simulink model "BlueROVHeavy_FeedbackLinearizationControl"  (R2024b)
settings: Solver=ode45  StartTime=0.0  StopTime=T  MaxStep=0.01  RelTol=1e-3
InitFcn:
  | run BlueRovHeavy_init.m;
StopFcn:
  | run BlueRovHeavy_plotting.m;
values from neighbouring files (symbols this model uses):
  BLUEROV_DATA = struct()    [BlueRovHeavy_data.m]
  Kf_D = 43    [BlueRovHeavy_init.m]
  Kf_P = 78    [BlueRovHeavy_init.m]
libraries: robotcorelib x1
settings Model: Creator=salva  LastModifiedBy=salva

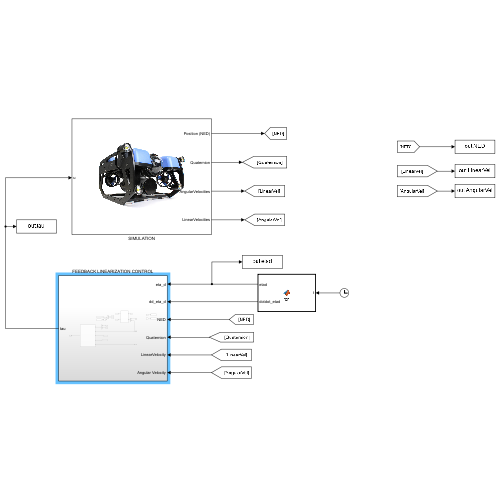
[thumbnail: Simulink's stored preview of the top-level diagram]
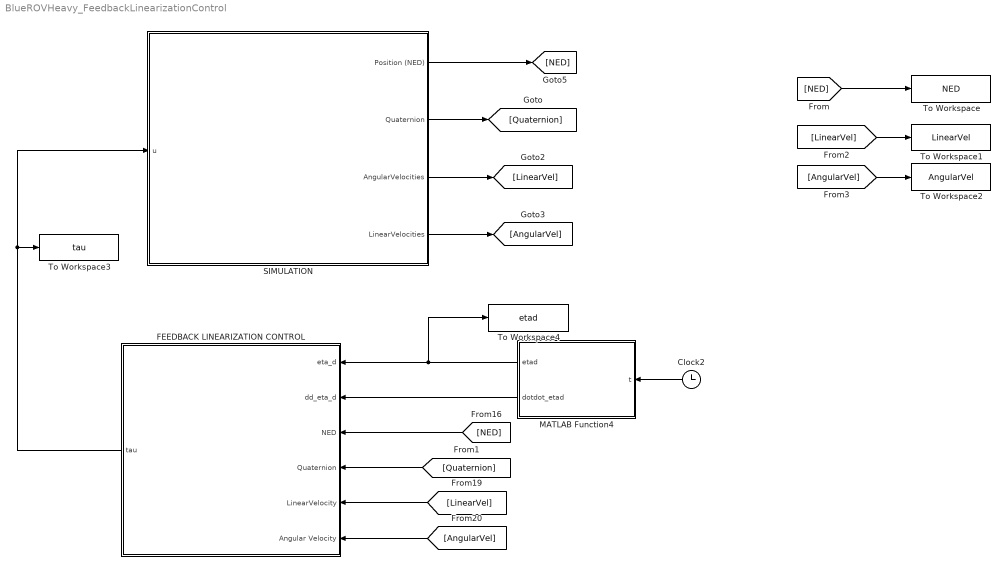
== system BlueROVHeavy_FeedbackLinearizationControl ==
  Clock2 : Clock
  FEEDBACK LINEARIZATION CONTROL : Subsystem
  MATLAB Function4 : MATLAB Function  TreatAsAtomicUnit=on
  SIMULATION : Subsystem
      mask Display: image('BlueROVpic.jpg', [0,0,0,0,90,90]);
  To Workspace : ToWorkspace  VariableName=NED  SaveFormat=Timeseries  SampleTime=-1
  To Workspace1 : ToWorkspace  VariableName=LinearVel  SaveFormat=Timeseries  SampleTime=-1
  To Workspace2 : ToWorkspace  VariableName=AngularVel  SaveFormat=Timeseries  SampleTime=-1
  To Workspace3 : ToWorkspace  VariableName=tau  SaveFormat=Timeseries  SampleTime=-1
  To Workspace4 : ToWorkspace  VariableName=etad  SaveFormat=Timeseries  SampleTime=-1
  wires:
  SIMULATION/1(Position (NED)) -> [NED]
  SIMULATION/2(Quaternion) -> [Quaternion]
  SIMULATION/3(AngularVelocities) -> [LinearVel]
  SIMULATION/4(LinearVelocities) -> [AngularVel]
  Clock2/1 -> MATLAB Function4/1(t)
  [LinearVel] -> FEEDBACK LINEARIZATION CONTROL/5(LinearVelocity)
  [AngularVel] -> FEEDBACK LINEARIZATION CONTROL/6(Angular Velocity)
  [Quaternion] -> FEEDBACK LINEARIZATION CONTROL/4(Quaternion)
  FEEDBACK LINEARIZATION CONTROL/1(tau) -> SIMULATION/1(u), To Workspace3/1
  MATLAB Function4/1(etad) -> To Workspace4/1, FEEDBACK LINEARIZATION CONTROL/1(eta_d)
  [NED] -> FEEDBACK LINEARIZATION CONTROL/3(NED)
  MATLAB Function4/2(dotdot_etad) -> FEEDBACK LINEARIZATION CONTROL/2(dd_eta_d)
  [NED] -> To Workspace/1
  [LinearVel] -> To Workspace1/1
  [AngularVel] -> To Workspace2/1

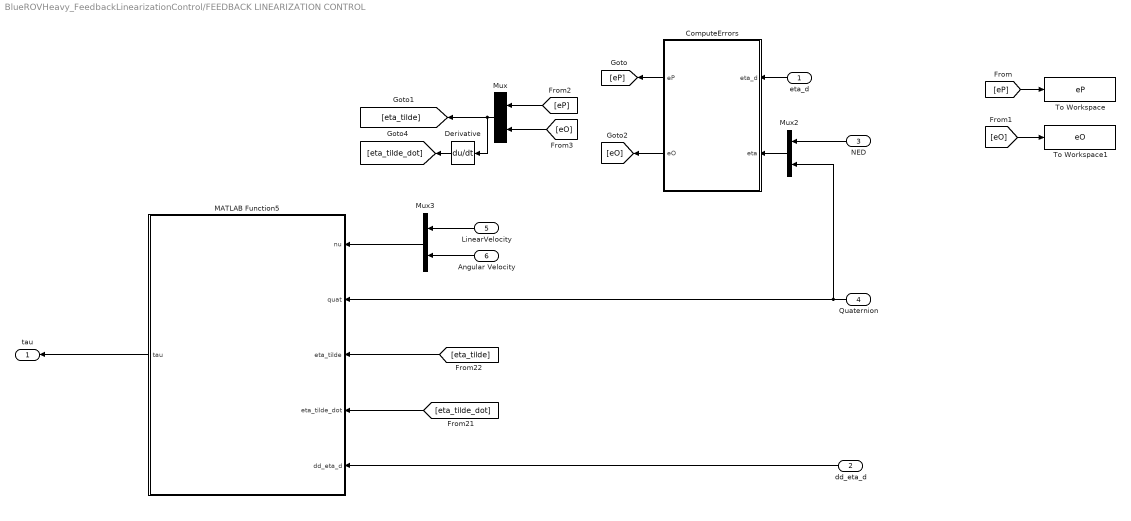
== system BlueROVHeavy_FeedbackLinearizationControl/FEEDBACK LINEARIZATION CONTROL ==
  eta_d : Inport
  dd_eta_d : Inport  Port=2
  NED : Inport  Port=3
  Quaternion : Inport  Port=4
  LinearVelocity : Inport  Port=5
  Angular Velocity : Inport  Port=6
  ComputeErrors : MATLAB Function  TreatAsAtomicUnit=on
  Derivative : Derivative
  MATLAB Function5 : MATLAB Function  TreatAsAtomicUnit=on
  Mux : Mux  Inputs=2
  Mux2 : Mux  Inputs=2
  Mux3 : Mux  Inputs=2
  To Workspace : ToWorkspace  VariableName=eP  SaveFormat=Timeseries  SampleTime=-1
  To Workspace1 : ToWorkspace  VariableName=eO  SaveFormat=Timeseries  SampleTime=-1
  tau : Outport
  wires:
  [eta_tilde_dot] -> MATLAB Function5/4(eta_tilde_dot)
  Mux2/1 -> ComputeErrors/2(eta)
  [eta_tilde] -> MATLAB Function5/3(eta_tilde)
  Mux3/1 -> MATLAB Function5/1(nu)
  LinearVelocity/1 -> Mux3/1
  Angular Velocity/1 -> Mux3/2
  MATLAB Function5/1(tau) -> tau/1
  NED/1 -> Mux2/1
  dd_eta_d/1 -> MATLAB Function5/5(dd_eta_d)
  eta_d/1 -> ComputeErrors/1(eta_d)
  Quaternion/1 -> MATLAB Function5/2(quat), Mux2/2
  Derivative/1 -> [eta_tilde_dot]
  Mux/1 -> [eta_tilde], Derivative/1
  ComputeErrors/1(eP) -> [eP]
  ComputeErrors/2(eO) -> [eO]
  [eP] -> To Workspace/1
  [eP] -> Mux/1
  [eO] -> Mux/2
  [eO] -> To Workspace1/1

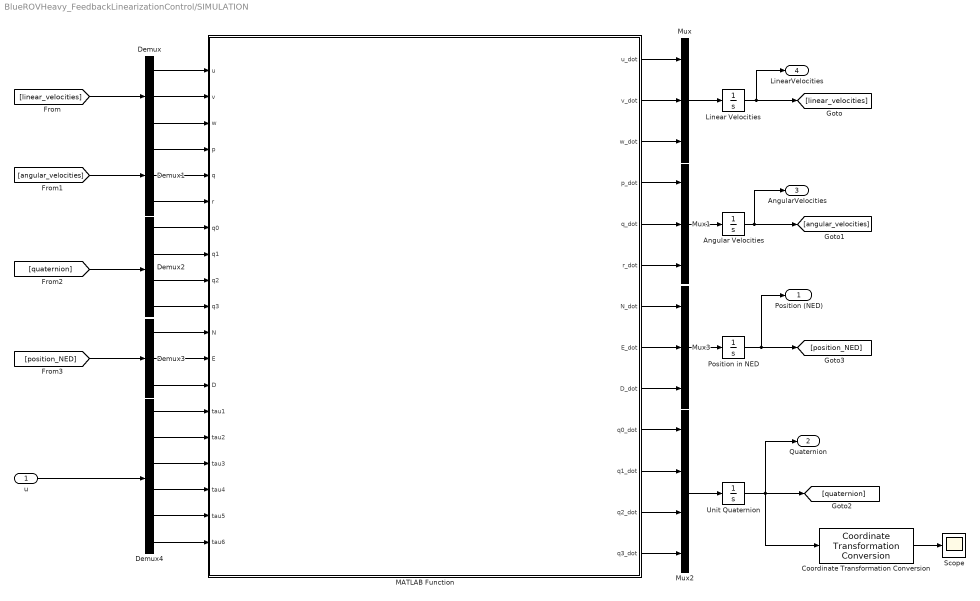
== system BlueROVHeavy_FeedbackLinearizationControl/SIMULATION ==
  u : Inport
  Angular Velocities : Integrator  InitialCondition=[0;0;0]  UpperSaturationLimit=50  LowerSaturationLimit=-50
  Coordinate Transformation Conversion : robotcorelib/Coordinate Transformation Conversion  InputRepresentation=Quaternion  InputEulerSequence=ZYX  ShowTrVecInputPort=on  OutputRepresentation=Euler Angles  OutputEulerSequence=XYZ  ShowTrVecOutputPort=on  SimulateUsing=Interpreted execution
  Demux : Demux  Outputs=3
  Demux1 : Demux  Outputs=3
  Demux2 : Demux
  Demux3 : Demux  Outputs=3
  Demux4 : Demux  Outputs=6
  Linear Velocities : Integrator  InitialCondition=[0.1;0;0]
  MATLAB Function : MATLAB Function  TreatAsAtomicUnit=on
  Mux : Mux  Inputs=3
  Mux1 : Mux  Inputs=3
  Mux2 : Mux
  Mux3 : Mux  Inputs=3
  Position in NED : Integrator  InitialCondition=[3.5;0;9.5]
  Scope : Scope
  Unit Quaternion : Integrator  InitialCondition=[1,0,0,0]
  Position (NED) : Outport
  Quaternion : Outport  Port=2
  AngularVelocities : Outport  Port=3
  LinearVelocities : Outport  Port=4
  wires:
  Demux/3 -> MATLAB Function/3(w)
  MATLAB Function/5(q_dot) -> Mux1/2
  Demux1/1 -> MATLAB Function/4(p)
  MATLAB Function/6(r_dot) -> Mux1/3
  Demux3/2 -> MATLAB Function/12(E)
  MATLAB Function/7(N_dot) -> Mux3/1
  Mux1/1 -> Angular Velocities/1
  Demux2/2 -> MATLAB Function/8(q1)
  MATLAB Function/2(v_dot) -> Mux/2
  Demux4/1 -> MATLAB Function/14(tau1)
  Demux3/3 -> MATLAB Function/13(D)
  Mux2/1 -> Unit Quaternion/1
  Demux4/4 -> MATLAB Function/17(tau4)
  Demux4/5 -> MATLAB Function/18(tau5)
  MATLAB Function/1(u_dot) -> Mux/1
  MATLAB Function/11(q1_dot) -> Mux2/2
  MATLAB Function/3(w_dot) -> Mux/3
  MATLAB Function/12(q2_dot) -> Mux2/3
  Demux3/1 -> MATLAB Function/11(N)
  MATLAB Function/4(p_dot) -> Mux1/1
  MATLAB Function/9(D_dot) -> Mux3/3
  [linear_velocities] -> Demux/1
  Demux4/3 -> MATLAB Function/16(tau3)
  u/1 -> Demux4/1
  Demux1/2 -> MATLAB Function/5(q)
  Mux/1 -> Linear Velocities/1
  Demux2/3 -> MATLAB Function/9(q2)
  [quaternion] -> Demux2/1
  Demux/1 -> MATLAB Function/1(u)
  Demux4/2 -> MATLAB Function/15(tau2)
  MATLAB Function/13(q3_dot) -> Mux2/4
  Demux2/4 -> MATLAB Function/10(q3)
  Mux3/1 -> Position in NED/1
  Demux2/1 -> MATLAB Function/7(q0)
  Unit Quaternion/1 -> Coordinate Transformation Conversion/1, Quaternion/1, [quaternion]
  Demux4/6 -> MATLAB Function/19(tau6)
  Position in NED/1 -> Position (NED)/1, [position_NED]
  Demux1/3 -> MATLAB Function/6(r)
  MATLAB Function/10(q0_dot) -> Mux2/1
  Angular Velocities/1 -> [angular_velocities], AngularVelocities/1
  [angular_velocities] -> Demux1/1
  Linear Velocities/1 -> [linear_velocities], LinearVelocities/1
  Demux/2 -> MATLAB Function/2(v)
  [position_NED] -> Demux3/1
  Coordinate Transformation Conversion/1 -> Scope/1
  MATLAB Function/8(E_dot) -> Mux3/2

== matlab function BlueROVHeavy_FeedbackLinearizationControl/FEEDBACK LINEARIZATION CONTROL/MATLAB Function5 ==
  data: nu input; tau output; quat input; eta_tilde input; eta_tilde_dot input; dd_eta_d input; BLUEROV_DATA parameter; Kf_D parameter; Kf_P parameter
function tau = fcn(nu,quat,eta_tilde,eta_tilde_dot,dd_eta_d, BLUEROV_DATA, Kf_D, Kf_P)

    u=nu(1);
    v=nu(2);
    w=nu(3);
    p=nu(4);
    q=nu(5);
    r=nu(6);
    q0=quat(1);
    q1=quat(2);
    q2=quat(3);
    q3=quat(4);




    % dq0=dotquat(1);
    % dq1=dotquat(2);
    % dq2=dotquat(3);
    % dq3=dotquat(4);
    Omega = 0.5 * [
     0   -p   -q  -r;
     p    0    r  -q;
     q  -r    0   p;
     r    q  -p   0
    ];

    dq= Omega*quat;
    dq0=dq(1);
    dq1=dq(2);
    dq2=dq(3);
    dq3=dq(4);





    e1 = BLUEROV_DATA.e1;                    %Body frame unit vector along x
    e2 = BLUEROV_DATA.e2;                    %Body frame unit vector along y
    e3 = BLUEROV_DATA.e3;                    %Body frame unit vector along z
    
    I3 = BLUEROV_DATA.I3;                      %Identity matrix (3x3)
    
    
    m_t = BLUEROV_DATA.m_t;                      %BlueROV mass [Kg]
    W = BLUEROV_DATA.W;                       %Weight [N]
    B = BLUEROV_DATA.B;                       %Boyancy [N]
    r_cb = BLUEROV_DATA.r_cb;                 %Center of boyancy wrt. center of origin [m]
    r_cg = BLUEROV_DATA.r_cg;                %Center of gravity wrt. center of origin [m]
    
    I = BLUEROV_DATA.I;                     %Dyadyic inertia
    SCG =BLUEROV_DATA.SCG;
    
    
    %% Added mass (hydrodynamic derivatives)
    
    X_udot = BLUEROV_DATA.X_udot;   % [kg] 
    Y_vdot = BLUEROV_DATA.Y_vdot;  % [kg]
    Z_wdot = BLUEROV_DATA.Z_wdot; % [kg]
    K_pdot = BLUEROV_DATA.K_pdot;  % [kg m^2/rad]
    M_qdot = BLUEROV_DATA.M_qdot;  % [kg m^2/rad]
    N_rdot = BLUEROV_DATA.N_rdot;  % [kg m^2/rad]
    
    %% Hydrodynamic linear and quadratic damping coefficients
    
    Xu = BLUEROV_DATA.Xu;      % [Ns/m]
    Yv = BLUEROV_DATA.Yv;      % [Ns/m]
    Zw = BLUEROV_DATA.Zw;      % [Ns/m]
    Kp = BLUEROV_DATA.Kp;      % [Ns/rad]
    Mq = BLUEROV_DATA.Mq;      % [Ns/rad]
    Nr = BLUEROV_DATA.Nr;      % [Ns/rad]
    
    Xuu = BLUEROV_DATA.Xuu;    % [Ns^2/m^2]
    Yvv = BLUEROV_DATA.Yvv;    % [Ns^2/m^2]
    Zww = BLUEROV_DATA.Zww;    % [Ns^2/m^2]
    Kpp = BLUEROV_DATA.Kpp;     % [Ns^2/rad^2]
    Mqq = BLUEROV_DATA.Mqq;     % [Ns^2/rad^2]
    Nrr = BLUEROV_DATA.Nrr;     % [Ns^2/rad^2]
        
    %% Kinematics
    
    Rq=[1-2*(q2^2+q3^2) 2*(q1*q2-q3*q0) 2*(q1*q3+q2*q0);
        2*(q1*q2+q3*q0) 1-2*(q1^2+q3^2) 2*(q2*q3-q1*q0);
        2*(q1*q3-q2*q0) 2*(q2*q3+q1*q0) 1-2*(q1^2+q2^2)];
    Tq=0.5*[-q1,-q2,-q3;
        q0,-q3,q2;
        q3,q0,-q1;
        -q2,q1,q0];

    J_qeta=[Rq,zeros(3,3);zeros(4,3),Tq];


 
    %% Computing Hydrodynamic Damping Matrix D(v)
    epsilon=1e-4;

    D = diag([Xu + Xuu*sqrt(u^2 + epsilon), ...
          Yv + Yvv*sqrt(v^2 + epsilon), ...
          Zw + Zww*sqrt(w^2 + epsilon), ...
          Kp + Kpp*sqrt(p^2 + epsilon), ...
          Mq + Mqq*sqrt(q^2 + epsilon), ...
          Nr + Nrr*sqrt(r^2 + epsilon)]);


    %% Computing Restoring Forces
    
    g_eta = [(-W+B)*(2*q1*q3-2*q2*q0);
            -(W-B)*(2*q2*q3-2*q1*q0);
            (W-B)*(2*q1^2+2*q2^2-1);
            r_cg(3)*W*(2*q2*q3+2*q1*q0);
            r_cg(3)*W*(2*q1*q3-2*q2*q0);
            0];
    
   
    %% Computing Coriolis and Centrifugal Matrix C(v)
     IO = I*[p q r]'; 
     
     S_IO = [0 -IO(3) IO(2);
             IO(3) 0 -IO(1);
            -IO(2) IO(1) 0]; 
             
    S_omega = [0 -r q;
              r 0 -p;
              -q p 0];         
             
       
    C_rb = [m_t*S_omega -m_t*S_omega*SCG;
            m_t*SCG*S_omega -S_IO];
        
    
    C_A = [0 0 0 0 -Z_wdot*w Y_vdot*v;
           0 0 0 -Z_wdot*w 0 -X_udot*u;
           0 0 0 -Y_vdot*v X_udot*u 0;
           0 -Z_wdot*w Y_vdot*v 0 -N_rdot*r M_qdot*q;
           Z_wdot*w 0 -X_udot*u N_rdot*r 0 -K_pdot*p;
           -Y_vdot*v X_udot*u 0 -M_qdot*q K_pdot*p 0];

    Cv=C_rb+C_A;

    %% Total Inertia
    M=BLUEROV_DATA.M;
    

    pinvJ_qeta=pinv(J_qeta); % Moonre_Penrose Inverse of the jacobian (since we are using quaternions)
    
    Jdot=compute_Jdot(q0,q1,q2,q3,dq0,dq1,dq2,dq3);%Jacobian derivative

    n=(Cv+D)*[u v w p q r]'+g_eta;

    lambda_n=dd_eta_d+Kf_D*eta_tilde_dot+Kf_P*eta_tilde;
    lambda_b=pinvJ_qeta*(lambda_n-Jdot*nu);

    tau=n+M*lambda_b;

== matlab function BlueROVHeavy_FeedbackLinearizationControl/SIMULATION/MATLAB Function ==
  data: u input; u_dot output; v input; w input; p input; q input; r input; q0 input; q1 input; q2 input; q3 input; N input; E input; D input; tau1 input; tau2 input; tau3 input; tau4 input; tau5 input; tau6 input; v_dot output; w_dot output; p_dot output; q_dot output; r_dot output; N_dot output; E_dot output; D_dot output; q0_dot output; q1_dot output; q2_dot output; q3_dot output; BLUEROV_DATA parameter

function [u_dot, v_dot, w_dot, p_dot, q_dot, r_dot,N_dot,E_dot,D_dot, q0_dot,q1_dot,q2_dot,q3_dot] =  ...
    BlueROV(u, v, w, p, q, r, q0,q1,q2,q3, N, E, D, tau1,tau2,tau3,tau4,tau5,tau6, BLUEROV_DATA)
    
    e1 = BLUEROV_DATA.e1;                    %Body frame unit vector along x
    e2 = BLUEROV_DATA.e2;                    %Body frame unit vector along y
    e3 = BLUEROV_DATA.e3;                    %Body frame unit vector along z
    
    I3 = BLUEROV_DATA.I3;                      %Identity matrix (3x3)
    
    
    m_t = BLUEROV_DATA.m_t;                      %BlueROV mass [Kg]
    W = BLUEROV_DATA.W;                       %Weight [N]
    B = BLUEROV_DATA.B;                       %Boyancy [N]
    r_cb = BLUEROV_DATA.r_cb;                 %Center of boyancy wrt. center of origin [m]
    r_cg = BLUEROV_DATA.r_cg;                %Center of gravity wrt. center of origin [m]
    
    I = BLUEROV_DATA.I;                     %Dyadyic inertia
    SCG =BLUEROV_DATA.SCG;
    
    
    %% Added mass (hydrodynamic derivatives)
    
    X_udot = BLUEROV_DATA.X_udot;   % [kg] 
    Y_vdot = BLUEROV_DATA.Y_vdot;  % [kg]
    Z_wdot = BLUEROV_DATA.Z_wdot; % [kg]
    K_pdot = BLUEROV_DATA.K_pdot;  % [kg m^2/rad]
    M_qdot = BLUEROV_DATA.M_qdot;  % [kg m^2/rad]
    N_rdot = BLUEROV_DATA.N_rdot;  % [kg m^2/rad]
    
    %% Hydrodynamic linear and quadratic damping coefficients
    
    Xu = BLUEROV_DATA.Xu;      % [Ns/m]
    Yv = BLUEROV_DATA.Yv;      % [Ns/m]
    Zw = BLUEROV_DATA.Zw;      % [Ns/m]
    Kp = BLUEROV_DATA.Kp;      % [Ns/rad]
    Mq = BLUEROV_DATA.Mq;      % [Ns/rad]
    Nr = BLUEROV_DATA.Nr;      % [Ns/rad]
    
    Xuu = BLUEROV_DATA.Xuu;    % [Ns^2/m^2]
    Yvv = BLUEROV_DATA.Yvv;    % [Ns^2/m^2]
    Zww = BLUEROV_DATA.Zww;    % [Ns^2/m^2]
    Kpp = BLUEROV_DATA.Kpp;     % [Ns^2/rad^2]
    Mqq = BLUEROV_DATA.Mqq;     % [Ns^2/rad^2]
    Nrr = BLUEROV_DATA.Nrr;     % [Ns^2/rad^2]
    
    
    
    %% Kinematics
    
    Rq=[1-2*(q2^2+q3^2) 2*(q1*q2-q3*q0) 2*(q1*q3+q2*q0);
        2*(q1*q2+q3*q0) 1-2*(q1^2+q3^2) 2*(q2*q3-q1*q0);
        2*(q1*q3-q2*q0) 2*(q2*q3+q1*q0) 1-2*(q1^2+q2^2)];
    Tq=0.5*[-q1,-q2,-q3;
        q0,-q3,q2;
        q3,q0,-q1;
        -q2,q1,q0];

    J_qeta=[Rq,zeros(3,3);zeros(4,3),Tq];
 
    %% Computing Hydrodynamic Damping Matrix D(v)
    epsilon=1e-4;

    D = diag([Xu + Xuu*sqrt(u^2 + epsilon), ...
          Yv + Yvv*sqrt(v^2 + epsilon), ...
          Zw + Zww*sqrt(w^2 + epsilon), ...
          Kp + Kpp*sqrt(p^2 + epsilon), ...
          Mq + Mqq*sqrt(q^2 + epsilon), ...
          Nr + Nrr*sqrt(r^2 + epsilon)]);


    %% Computing Restoring Forces
    
    g_eta = [(-W+B)*(2*q1*q3-2*q2*q0);
            -(W-B)*(2*q2*q3-2*q1*q0);
            (W-B)*(2*q1^2+2*q2^2-1);
            r_cg(3)*W*(2*q2*q3+2*q1*q0);
            r_cg(3)*W*(2*q1*q3-2*q2*q0);
            0];
    
   
    %% Computing Coriolis and Centrifugal Matrix C(v)
     IO = I*[p q r]'; 
     
     S_IO = [0 -IO(3) IO(2);
             IO(3) 0 -IO(1);
            -IO(2) IO(1) 0]; 
             
    S_omega = [0 -r q;
              r 0 -p;
              -q p 0];         
             
       
    C_rb = [m_t*S_omega -m_t*S_omega*SCG;
            m_t*SCG*S_omega -S_IO];
        
    
    C_A = [0 0 0 0 -Z_wdot*w Y_vdot*v;
           0 0 0 -Z_wdot*w 0 -X_udot*u;
           0 0 0 -Y_vdot*v X_udot*u 0;
           0 -Z_wdot*w Y_vdot*v 0 -N_rdot*r M_qdot*q;
           Z_wdot*w 0 -X_udot*u N_rdot*r 0 -K_pdot*p;
           -Y_vdot*v X_udot*u 0 -M_qdot*q K_pdot*p 0];
        
    %% Generalized forces and moments
    tau_c = [tau1 tau2 tau3 tau4 tau5 tau6]';

    %% Total Inertia Matric
    M=BLUEROV_DATA.M;


    %% 6DOF Dynamics and Kinematics
    
    nu_dot=zeros(6,1);
    nu_dot = M\(tau_c-(D+C_rb+C_A)*[u v w p q r]' -g_eta); %6DOF dynamics

    etadot=zeros(7,1); 
    etadot=J_qeta*[u v w p q r]'; %Kinematics
    
    u_dot = nu_dot(1); %Surge velcoity
    v_dot = nu_dot(2); %Sway Velcoity
    w_dot = nu_dot(3); %Heave velocity
    p_dot = nu_dot(4); %Angular velocity around phi
    q_dot = nu_dot(5);  %Angular velcoity around theta
    r_dot = nu_dot(6); %Angular velcoity around psi
  
   
    
    N_dot=etadot(1); % N position
    E_dot=etadot(2); % E position
    D_dot=etadot(3); % D position
    q0_dot=etadot(4); % Quaternion
    q1_dot=etadot(5);
    q2_dot=etadot(6);
    q3_dot=etadot(7);

== matlab function BlueROVHeavy_FeedbackLinearizationControl/FEEDBACK LINEARIZATION CONTROL/ComputeErrors ==
  data: eP output; eta_d input; eO output; eta input
function [eP,eO] = fcn(eta_d,eta)

Qd=eta_d(4:7);
Qe=eta(4:7);

Sd=[0 -Qd(4) Qd(3);
    Qd(4) 0 -Qd(2);
    -Qd(3) Qd(2) 0];

eO=[Qd(1)*Qe(1)+Qd(2:4)'*Qe(2:4);Qe(1)*Qd(2:4)-Qd(1)*Qe(2:4)-Sd*Qe(2:4)];

eP=eta_d(1:3)-eta(1:3);

== matlab function BlueROVHeavy_FeedbackLinearizationControl/MATLAB Function4 ==
  data: t input; etad output; dotdot_etad output
function [etad,dotdot_etad]  = fcn(t)
% Traiettoria elicoidale 3D con quaternione costante
% etad = [x, y, z, qx, qy, qz, qw]'
% dot_etad = derivata prima
% dotdot_etad = derivata seconda

% Parametri della spirale
r = 4;         % Raggio dell'elica
omega = 0.8;  % Frequenza angolare (rad/s)
vz = 0.6;      % Velocità lungo z

% Posizione elicoidale
x = r * cos(omega * t);
y = r * sin(omega * t);
z = 10+vz * t;

% Derivata prima della posizione
dx = -r * omega * sin(omega * t);
dy =  r * omega * cos(omega * t);
dz = vz;

% Derivata seconda della posizione
ddx = -r * omega^2 * cos(omega * t);
ddy = -r * omega^2 * sin(omega * t);
ddz = 0;

% Quaternione costante (nessuna rotazione)
qx = 1;
qy = 0;
qz = 0;
qw = 0;

% Stato desiderato
etad = [x; y; z; qx; qy; qz; qw];

% Derivata seconda
dotdot_etad = [ddx; ddy; ddz; 0; 0; 0; 0];

end
